simulink model "postProcessing"  (R2019a)
settings: Solver=VariableStepAuto  StartTime=0.0  StopTime=10.0  RelTol=1e-3
settings Model: LastModifiedBy=dq16394
settings ModelReferenceCC: ModelReferenceNumInstancesAllowed=Single

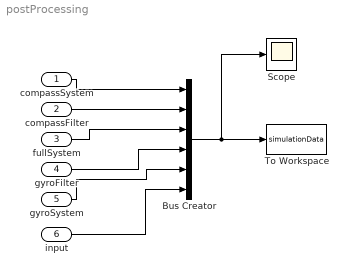
== system postProcessing ==
  compassSystem : Inport
  compassFilter : Inport  Port=2
  fullSystem : Inport  Port=3
  gyroFilter : Inport  Port=4
  gyroSystem : Inport  Port=5
  input : Inport  Port=6
  Bus Creator : BusCreator  Inputs=6
  Scope : Scope
  To Workspace : ToWorkspace  VariableName=simulationData  SaveFormat=Structure With Time  SampleTime=-1
  wires:
  fullSystem/1 -> Bus Creator/3
  compassSystem/1 -> Bus Creator/1
  compassFilter/1 -> Bus Creator/2
  input/1 -> Bus Creator/6
  Bus Creator/1 -> To Workspace/1, Scope/1
  gyroFilter/1 -> Bus Creator/4
  gyroSystem/1 -> Bus Creator/5
